simulink model "r2bb2xpfb14mcr23"  (R2012b)
settings: Solver=VariableStepDiscrete  SolverMode=SingleTasking  StartTime=0.0  StopTime=10.0  RelTol=1e-3
undefined symbols (not defined in the file): bit_reverse, pfb_coeff_gen_calc
libraries: xbsIndex_r4 x7733, casper_library_misc x51, casper_library_delays x18, xps_library x5
(part 15 of 103)

== system r2bb2xpfb14mcr23/fft_biplex_2by2_real/fft_biplex_real_2x2/bi_real_unscr_2x ==
  sync : Inport
  even : Inport  Port=2
  odd : Inport  Port=3
  constant : xbsIndex_r4/Constant  const=0  gui_display_data_type=Fixed-point  arith_type=Unsigned  n_bits=13  bin_pt=0  preci_type=Single  exp_width=8  frac_width=24  explicit_period=on  period=1  equ=P=C  opselect=C  inp2=PCIN>>17  opr=+  inp1=P  carry=CIN  dbl_ovrd=off  block_type=constant
  count : xbsIndex_r4/Counter  cnt_type=Free Running  cnt_to=Inf  operation=Up  start_count=0  cnt_by_val=1  arith_type=Unsigned  n_bits=13  bin_pt=0  load_pin=off  rst=on  en=off  explicit_period=on  period=1  dbl_ovrd=off  use_behavioral_HDL=on  implementation=Fabric  block_type=counter
  d0 : xbsIndex_r4/Delay  rst=off  infoeditControl=Selection of Reset will increase slice count due to use of real FFs and instead of SRLs  en=off  latency=1  dbl_ovrd=off  reg_retiming=on  block_type=delay
  en_even : xbsIndex_r4/Constant  const=1  gui_display_data_type=Fixed-point  arith_type=Boolean  n_bits=1  bin_pt=0  preci_type=Single  exp_width=8  frac_width=24  explicit_period=on  period=1  equ=P=C  opselect=C  inp2=PCIN>>17  opr=+  inp1=P  carry=CIN  dbl_ovrd=off  block_type=constant
  en_odd : xbsIndex_r4/Constant  const=1  gui_display_data_type=Fixed-point  arith_type=Boolean  n_bits=1  bin_pt=0  preci_type=Single  exp_width=8  frac_width=24  explicit_period=on  period=1  equ=P=C  opselect=C  inp2=PCIN>>17  opr=+  inp1=P  carry=CIN  dbl_ovrd=off  block_type=constant
  even_delay : xbsIndex_r4/Delay  rst=off  infoeditControl=Selection of Reset will increase slice count due to use of real FFs and instead of SRLs  en=off  latency=1  dbl_ovrd=off  reg_retiming=on  block_type=delay
  hilbert : Subsystem  AncestorBlock=casper_library_ffts_internal/hilbert  mask(hilbert){n_inputs=1, BitWidth=n_bits, bin_pt_in=bin_pt, add_latency=add_latency, conv_latency=conv_latency, misc=off}
      mask prompts: n_inputs "Number simultaneous inputs"; BitWidth "Bit Width"; bin_pt_in "Binary point in"; add_latency "Add Latency"; conv_latency "Convert Latency"; misc "Miscellaneous input"
      mask help:
      | FFT internal block.
      |
      | Computes (a+b*)/2 and (a-b*)/2i.
      |
      | If a = w + ix and b = y + iz, then:
      | a+b = (w+y)/2 + i(x-z)/2
      | a-b = (x+z)/2 + i(y-w)/2
      mask init:
      | hilbert_init(gcb, ...
      |     'n_inputs', n_inputs, ...
      |     'BitWidth', BitWidth, ...
      |     'bin_pt_in', bin_pt_in, ...
      |     'add_latency', add_latency, ...
      |     'conv_latency', conv_latency, ...
      |     'misc', misc);
  mux : xbsIndex_r4/Mux  inputs=2  en=off  latency=1  precision=Full  arith_type=Unsigned  n_bits=16  bin_pt=14  quantization=Truncate  overflow=Wrap  dbl_ovrd=off  block_type=mux
  relational : xbsIndex_r4/Relational  mode=a=b  en=off  latency=0  dbl_ovrd=off  block_type=relational
  reorder_even : Subsystem  AncestorBlock=casper_library_reorder/reorder  mask(reorder){map=[0 4096 2048 6144 1024 5120 3072 7168 512 4608 2560 6656 1536 5632 3584 7680 256 4352 2304 6400 1280 5376 3328 7424 768 4864 2816 6912 1792 5888 3840 7936 128 4224 2176 6272 1152 5248 3200 7296 640 4736 2688 6784 1664 5760 3712 7808 384 4480 2432 6528 1408 5504 3456 7552 896 4992 2944 7040 1920 6016 3968 8064 64 4160 2112 6208 1088 5184 3136 7232 576 4672 2624 6720 1600 5696 3648 7744 320 4416 2368 6464 1344 5440 3392 7488 832 4928 2880 6976 1856 5952 3904 8000 192 4288 2240 6336 1216 5312 3264 7360 704 4800 2752 6848 1728 5824 3776 7872 448 4544 2496 6592 1472 5568 3520 7616 960 5056 3008 7104 1984 6080 4032 8128 32 4128 2080 6176 1056 5152 3104 7200 544 4640 2592 6688 1568 5664 3616 7712 288 4384 2336 6432 1312 5408 3360 7456 800 4896 2848 6944 1824 5920 3872 7968 160 4256 2208 6304 1184 5280 3232 7328 672 4768 2720 6816 1696 5792 3744 7840 416 4512 2464 6560 1440 5536 3488 7584 928 5024 2976 7072 1952 6048 4000 8096 96 4192 2144 6240 1120 5216 3168 7264 608 4704 2656 6752 1632 5728 3680 7776 352 4448 2400 6496 1376 5472 3424 7520 864 4960 2912 7008 1888 5984 3936 8032 224 4320 2272 6368 1248 5344 3296 7392 736 4832 2784 6880 1760 5856 3808 7904 480 4576 2528 6624 1504 5600 3552 7648 992 5088 3040 7136 2016 6112 4064 8160 16 4112 2064 6160 1040 5136 3088 7184 528 4624 2576 6672 1552 5648 3600 7696 272 4368 2320 6416 1296 5392 3344 7440 784 4880 2832 6928 1808 5904 3856 7952 144 4240 2192 6288 1168 5264 3216 7312 656 4752 2704 6800 1680 5776 3728 7824 400 4496 2448 6544 1424 5520 3472 7568 912 5008 2960 7056 1936 6032 3984 8080 80 4176 2128 6224 1104 5200 3152 7248 592 4688 2640 6736 1616 5712 3664 7760 336 4432 2384 6480 1360 5456 3408 7504 848 4944 2896 6992 1872 5968 3920 8016 208 4304 2256 6352 1232 5328 3280 7376 720 4816 2768 6864 1744 5840 3792 7888 464 4560 2512 6608 1488 5584 3536 7632 976 5072 3024 7120 2000 6096 4048 8144 48 4144 2096 6192 1072 5168 3120 7216 560 4656 2608 6704 1584 5680 3632 7728 304 4400 2352 6448 1328 5424 3376 7472 816 4912 2864 6960 1840 5936 3888 7984 176 4272 2224 6320 1200 5296 3248 7344 688 4784 2736 6832 1712 5808 3760 7856 432 4528 2480 6576 1456 5552 3504 7600 944 5040 2992 7088 1968 6064 4016 8112 112 4208 2160 6256 1136 5232 3184 7280 624 4720 2672 6768 1648 5744 3696 7792 368 4464 2416 6512 1392 5488 3440 7536 880 4976 2928 7024 1904 6000 3952 8048 240 4336 2288 6384 1264 5360 3312 7408 752 4848 2800 6896 1776 5872 3824 7920 496 4592 2544 6640 1520 5616 3568 7664 1008 5104 3056 7152 2032 6128 4080 8176 8 4104 2056 6152 1032 5128 3080 7176 520 4616 2568 6664 1544 5640 3592 7688 264 4360 2312 6408 1288 5384 3336 7432 776 4872 2824 6920 1800 5896 3848 7944 136 4232 2184 6280 1160 5256 3208 7304 648 4744 2696 6792 1672 5768 3720 7816 392 4488 2440 6536 1416 5512 3464 7560 904 5000 2952 7048 1928 6024 3976 8072 72 4168 2120 6216 1096 5192 3144 7240 584 4680 2632 6728 1608 5704 3656 7752 328 4424 2376 6472 1352 5448 3400 7496 840 4936 2888 6984 1864 5960 3912 8008 200 4296 2248 6344 1224 5320 3272 7368 712 4808 2760 6856 1736 5832 3784 7880 456 4552 2504 6600 1480 5576 3528 7624 968 5064 3016 7112 1992 6088 4040 8136 40 4136 2088 6184 1064 5160 3112 7208 552 4648 2600 6696 1576 5672 3624 7720 296 4392 2344 6440 1320 5416 3368 7464 808 4904 2856 6952 1832 5928 3880 7976 168 4264 2216 6312 1192 5288 3240 7336 680 4776 2728 6824 1704 5800 3752 7848 424 4520 2472 6568 1448 5544 3496 7592 936 5032 2984 7080 1960 6056 4008 8104 104 4200 2152 6248 1128 5224 3176 7272 616 4712 2664 6760 1640 5736 3688 7784 360 4456 2408 6504 1384 5480 3432 7528 872 4968 2920 7016 1896 5992 3944 8040 232 4328 2280 6376 1256 5352 3304 7400 744 4840 2792 6888 1768 5864 3816 7912 488 4584 2536 6632 1512 5608 3560 7656 1000 5096 3048 7144 2024 6120 4072 8168 24 4120 2072 6168 1048 5144 3096 7192 536 4632 2584 6680 1560 5656 3608 7704 280 4376 2328 6424 1304 5400 3352 7448 792 4888 2840 6936 1816 5912 3864 7960 152 4248 2200 6296 1176 5272 3224 7320 664 4760 2712 6808 1688 5784 3736 7832 408 4504 2456 6552 1432 5528 ...(+35854 chars)], n_bits=0, n_inputs=1, bram_latency=2, map_latency=1, fanout_latency=0, double_buffer=0, bram_map=on}
      mask prompts: map "Output Order:"; n_bits "Data width in"; n_inputs "Number of inputs"; bram_latency "BRAM Latency"; map_latency "Map Latency"; fanout_latency "Fanout latency"; double_buffer "Double Buffer"; bram_map "Use BlockRAM for Map"
      mask init:
      | reorder_init(gcb, ...
      |     'map', map, ...
      |     'n_bits', n_bits, ...
      |     'n_inputs', n_inputs, ...
      |     'bram_latency', bram_latency, ...
      |     'map_latency', map_latency, ...
      |     'fanout_latency', fanout_latency, ...
      |     'double_buffer', double_buffer, ...
      |     'bram_map', bram_map);
      settings: AttributesFormatString=order=2
      mask Help: eval('xlWeb(''http://casper.berkeley.edu/wiki/Reorder'')')
  reorder_odd : Subsystem  AncestorBlock=casper_library_reorder/reorder  mask(reorder){map=[8191 4095 6143 2047 7167 3071 5119 1023 7679 3583 5631 1535 6655 2559 4607 511 7935 3839 5887 1791 6911 2815 4863 767 7423 3327 5375 1279 6399 2303 4351 255 8063 3967 6015 1919 7039 2943 4991 895 7551 3455 5503 1407 6527 2431 4479 383 7807 3711 5759 1663 6783 2687 4735 639 7295 3199 5247 1151 6271 2175 4223 127 8127 4031 6079 1983 7103 3007 5055 959 7615 3519 5567 1471 6591 2495 4543 447 7871 3775 5823 1727 6847 2751 4799 703 7359 3263 5311 1215 6335 2239 4287 191 7999 3903 5951 1855 6975 2879 4927 831 7487 3391 5439 1343 6463 2367 4415 319 7743 3647 5695 1599 6719 2623 4671 575 7231 3135 5183 1087 6207 2111 4159 63 8159 4063 6111 2015 7135 3039 5087 991 7647 3551 5599 1503 6623 2527 4575 479 7903 3807 5855 1759 6879 2783 4831 735 7391 3295 5343 1247 6367 2271 4319 223 8031 3935 5983 1887 7007 2911 4959 863 7519 3423 5471 1375 6495 2399 4447 351 7775 3679 5727 1631 6751 2655 4703 607 7263 3167 5215 1119 6239 2143 4191 95 8095 3999 6047 1951 7071 2975 5023 927 7583 3487 5535 1439 6559 2463 4511 415 7839 3743 5791 1695 6815 2719 4767 671 7327 3231 5279 1183 6303 2207 4255 159 7967 3871 5919 1823 6943 2847 4895 799 7455 3359 5407 1311 6431 2335 4383 287 7711 3615 5663 1567 6687 2591 4639 543 7199 3103 5151 1055 6175 2079 4127 31 8175 4079 6127 2031 7151 3055 5103 1007 7663 3567 5615 1519 6639 2543 4591 495 7919 3823 5871 1775 6895 2799 4847 751 7407 3311 5359 1263 6383 2287 4335 239 8047 3951 5999 1903 7023 2927 4975 879 7535 3439 5487 1391 6511 2415 4463 367 7791 3695 5743 1647 6767 2671 4719 623 7279 3183 5231 1135 6255 2159 4207 111 8111 4015 6063 1967 7087 2991 5039 943 7599 3503 5551 1455 6575 2479 4527 431 7855 3759 5807 1711 6831 2735 4783 687 7343 3247 5295 1199 6319 2223 4271 175 7983 3887 5935 1839 6959 2863 4911 815 7471 3375 5423 1327 6447 2351 4399 303 7727 3631 5679 1583 6703 2607 4655 559 7215 3119 5167 1071 6191 2095 4143 47 8143 4047 6095 1999 7119 3023 5071 975 7631 3535 5583 1487 6607 2511 4559 463 7887 3791 5839 1743 6863 2767 4815 719 7375 3279 5327 1231 6351 2255 4303 207 8015 3919 5967 1871 6991 2895 4943 847 7503 3407 5455 1359 6479 2383 4431 335 7759 3663 5711 1615 6735 2639 4687 591 7247 3151 5199 1103 6223 2127 4175 79 8079 3983 6031 1935 7055 2959 5007 911 7567 3471 5519 1423 6543 2447 4495 399 7823 3727 5775 1679 6799 2703 4751 655 7311 3215 5263 1167 6287 2191 4239 143 7951 3855 5903 1807 6927 2831 4879 783 7439 3343 5391 1295 6415 2319 4367 271 7695 3599 5647 1551 6671 2575 4623 527 7183 3087 5135 1039 6159 2063 4111 15 8183 4087 6135 2039 7159 3063 5111 1015 7671 3575 5623 1527 6647 2551 4599 503 7927 3831 5879 1783 6903 2807 4855 759 7415 3319 5367 1271 6391 2295 4343 247 8055 3959 6007 1911 7031 2935 4983 887 7543 3447 5495 1399 6519 2423 4471 375 7799 3703 5751 1655 6775 2679 4727 631 7287 3191 5239 1143 6263 2167 4215 119 8119 4023 6071 1975 7095 2999 5047 951 7607 3511 5559 1463 6583 2487 4535 439 7863 3767 5815 1719 6839 2743 4791 695 7351 3255 5303 1207 6327 2231 4279 183 7991 3895 5943 1847 6967 2871 4919 823 7479 3383 5431 1335 6455 2359 4407 311 7735 3639 5687 1591 6711 2615 4663 567 7223 3127 5175 1079 6199 2103 4151 55 8151 4055 6103 2007 7127 3031 5079 983 7639 3543 5591 1495 6615 2519 4567 471 7895 3799 5847 1751 6871 2775 4823 727 7383 3287 5335 1239 6359 2263 4311 215 8023 3927 5975 1879 6999 2903 4951 855 7511 3415 5463 1367 6487 2391 4439 343 7767 3671 5719 1623 6743 2647 4695 599 7255 3159 5207 1111 6231 2135 4183 87 8087 3991 6039 1943 7063 2967 5015 919 7575 3479 5527 1431 6551 2455 4503 407 7831 3735 5783 1687 6807 2711 4759 663 7319 3223 5271 1175 6295 2199 4247 151 7959 3863 5911 1815 6935 2839 4887 791 7447 3351 5399 1303 6423 2327 4375 279 7703 3607 5655 1559 6679 2583 4631 535 7191 3095 5143 1047 6167 2071 4119 23 8167 4071 6119 2023 7143 3047 5095 999 7655 3559 5607 1511 6631 2535 4583 487 7911 3815 5863 1767 6887 2791 4839 743 7399 3303 5351 1255 6375 2279 4327 231 8039 3943 5991 1895 7015 2919 4967 871 7527 3431 5479 1383 6503 2407 4455 359 7783 3687 5735 1639 6759 ...(+35853 chars)], n_bits=0, n_inputs=1, bram_latency=2, map_latency=1, fanout_latency=0, double_buffer=0, bram_map=on}
      mask prompts: map "Output Order:"; n_bits "Data width in"; n_inputs "Number of inputs"; bram_latency "BRAM Latency"; map_latency "Map Latency"; fanout_latency "Fanout latency"; double_buffer "Double Buffer"; bram_map "Use BlockRAM for Map"
      mask init: same as r2bb2xpfb14mcr23/fft_biplex_2by2_real/fft_biplex_real_2x2/bi_real_unscr_2x/reorder_even
      settings: AttributesFormatString=order=2
      mask Help: eval('xlWeb(''http://casper.berkeley.edu/wiki/Reorder'')')
  sync_delay : xbsIndex_r4/Delay  rst=off  infoeditControl=Selection of Reset will increase slice count due to use of real FFs and instead of SRLs  en=off  latency=add_latency + conv_latency + 1  dbl_ovrd=off  reg_retiming=on  block_type=delay
  t0 : Terminator
  t1 : Terminator
  t2 : Terminator
  sync_out : Outport
  pol13_out : Outport  Port=2
  pol24_out : Outport  Port=3
  wires:
  sync/1 -> reorder_even/1(sync), reorder_odd/1(sync)
  even/1 -> reorder_even/3(din0)
  odd/1 -> reorder_odd/3(din0)
  en_even/1 -> reorder_even/2(en)
  en_odd/1 -> reorder_odd/2(en)
  reorder_even/2(valid) -> t0/1
  reorder_odd/1(sync_out) -> t1/1
  reorder_odd/2(valid) -> t2/1
  reorder_even/1(sync_out) -> count/1, sync_delay/1
  count/1 -> relational/1
  constant/1 -> relational/2
  reorder_odd/3(dout0) -> d0/1
  relational/1 -> mux/1
  reorder_even/3(dout0) -> mux/3, even_delay/1
  d0/1 -> mux/2
  sync_delay/1 -> sync_out/1
  even_delay/1 -> hilbert/1(a)
  mux/1 -> hilbert/2(b)
  hilbert/1(even) -> pol13_out/1
  hilbert/2(odd) -> pol24_out/1
